simulink subsystem "pd_plus_controller_refsys"  (R2022b)
settings: Solver=VariableStepAuto  StartTime=0.0  StopTime=10.0  RelTol=1e-3
settings Model: Creator=emu  LastModifiedBy=emu

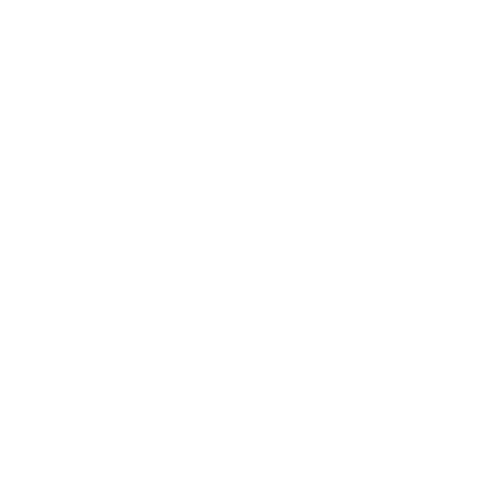
[thumbnail: Simulink's stored preview of the top-level diagram]
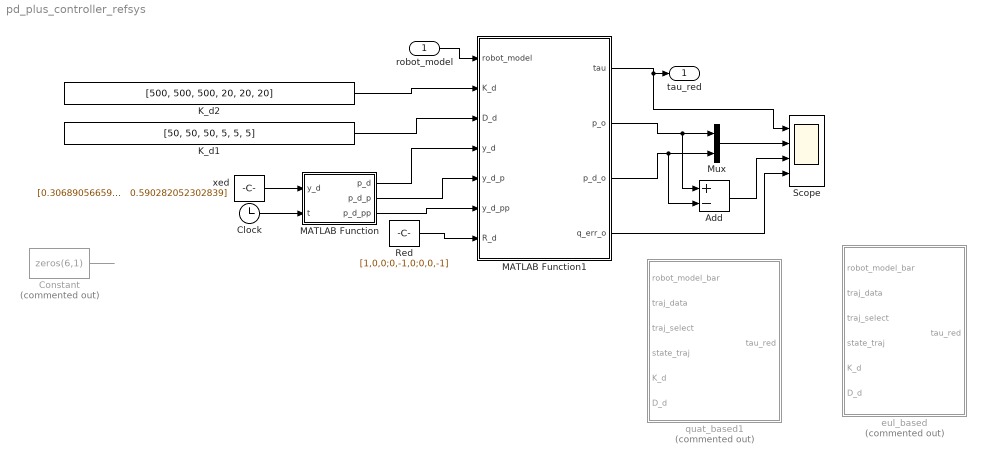
== system pd_plus_controller_refsys ==
  robot_model : Inport  OutDataTypeStr=Bus: robot_model_red
  Add : Sum  Inputs=+-
  Clock : Clock
  Constant : Constant  Commented=on  Value=zeros(6,1)
  K_d1 : Constant  Value=[50, 50, 50, 5, 5, 5]
  K_d2 : Constant  Value=[500, 500, 500, 20, 20, 20]
  MATLAB Function : MATLAB Function  TreatAsAtomicUnit=on
  MATLAB Function1 : MATLAB Function  TreatAsAtomicUnit=on
  Mux : Mux  Inputs=2
  Red : Constant  Value=[1,0,0;0,-1,0;0,0,-1]
  Scope : Scope  NumInputPorts=4
  eul_based : MATLAB Function  Commented=on  TreatAsAtomicUnit=on
  quat_based1 : MATLAB Function  Commented=on  TreatAsAtomicUnit=on
  xed : Constant  Value="[0.306890566592941  -0.000000000000000   0.590282052302839]"
  tau_red : Outport
  wires:
  robot_model/1 -> MATLAB Function1/1(robot_model)
  MATLAB Function1/1(tau) -> tau_red/1, Scope/1
  K_d2/1 -> MATLAB Function1/2(K_d)
  K_d1/1 -> MATLAB Function1/3(D_d)
  MATLAB Function/1(p_d) -> MATLAB Function1/4(y_d)
  Constant/1 -> ?
  MATLAB Function1/4(q_err_o) -> Scope/4
  Mux/1 -> Scope/2
  MATLAB Function1/2(p_o) -> Mux/1, Add/1
  MATLAB Function1/3(p_d_o) -> Mux/2, Add/2
  Clock/1 -> MATLAB Function/2(t)
  Red/1 -> MATLAB Function1/7(R_d)
  xed/1 -> MATLAB Function/1(y_d)
  MATLAB Function/2(p_d_p) -> MATLAB Function1/5(y_d_p)
  MATLAB Function/3(p_d_pp) -> MATLAB Function1/6(y_d_pp)
  Add/1 -> Scope/3

== matlab function pd_plus_controller_refsys/MATLAB Function ==
  data: y_d input; p_d output; t input; p_d_p output; p_d_pp output
function [p_d, p_d_p, p_d_pp] = fcn(y_d, t)

omega=0.1;
f = cos(omega*t);
df = -omega*sin(omega*t);
ddf = -omega^2 * cos(omega*t);

a=0.2;
p_d = [y_d(1); -0.2+y_d(2)+a*f; y_d(3)];
p_d_p = [0; a*df; 0];
p_d_pp = [0; a*ddf; 0];

== matlab function pd_plus_controller_refsys/MATLAB Function1 ==
  data: robot_model input Bus: robot_model_red; tau output; K_d input; D_d input; y_d input; y_d_p input; y_d_pp input; p_o output; p_d_o output; q_err_o output; R_d input
function [tau, p_o, p_d_o, q_err_o] = fcn(robot_model, K_d, D_d, y_d, y_d_p, y_d_pp, R_d)

M = robot_model.M;
C_rnea = robot_model.C_rnea;
J = robot_model.J;
J_p = robot_model.J_p;
H = robot_model.H;

q = robot_model.q;
q_p = robot_model.q_p;

% Desired Trajectory
p_d    = y_d;
p_d_p  = y_d_p;
p_d_pp = y_d_pp;

omega_d = zeros(3,1);
omega_d_p = zeros(3,1);

% Actual Sizes
x_p = J * q_p;
R = H(1:3,1:3);

p = H(1:3,4);
p_p = x_p(1:3);

omega = x_p(4:6); % Drehwinkelgeschwindigkeit des Endeffektors

% Errors
RR = R_d'*R;
q_err_tmp   = rotm2quat_v4(RR);
epsilon = q_err_tmp(2:4);
eta = q_err_tmp(1);
q_err = 2 * R_d * (eta * eye(3) + skew(epsilon)) * (K_d(4:6) .* epsilon);

x_err   = [K_d(1:3) .* (p-p_d); q_err];   % Error as quaternion
x_err_p = [p_p-p_d_p;  omega-omega_d];
x_d_pp  = [p_d_pp;     omega_d_p];

J_sym = J * J' + 1e-6*eye(6);
J_sym2 = 1/2 * (J_sym + J_sym');
J_pinv = J'/J_sym2;

tau = C_rnea + M*J_pinv*(x_d_pp - J_p*q_p) - J' * (D_d .* x_err_p + x_err);

p_o = p;
p_d_o = p_d;
q_err_o = q_err;

== matlab function pd_plus_controller_refsys/quat_based1 ==
  data: robot_model_bar input; tau_red output; traj_data input Bus: traj_data_bus; traj_select input; state_traj input Bus: state_traj_bus; K_d input; D_d input; param_robot parameter
function tau_red = fcn(robot_model_bar, traj_data, traj_select, state_traj, K_d, D_d, param_robot)

persistent cnt;
persistent run_flag;

if(isempty(cnt))
    cnt = 1;
    run_flag = 0;
end

%cnt = 1; % ignore cnt;

n_red = param_robot.n_red;
n_indices = param_robot.n_indices;

q_bar = robot_model_bar.q;
q_p_bar = robot_model_bar.q_p;

M_bar = robot_model_bar.M;
C_bar = robot_model_bar.C;
J_bar = robot_model_bar.J;
J_p_bar = robot_model_bar.J_p;
H_bar = robot_model_bar.H;

M_red = M_bar(n_indices, n_indices);
C_red = C_bar(n_indices, n_indices);
J_red = J_bar(:, n_indices);
J_p_red = J_p_bar(:, n_indices);

q_red = q_bar(n_indices);
q_p_red = q_p_bar(n_indices);

% Desired Trajectory
p_d    = traj_data.p_d(:, cnt, traj_select);
p_d_p  = traj_data.p_d_p(:, cnt, traj_select);
p_d_pp = traj_data.p_d_pp(:, cnt, traj_select);

R_d = traj_data.R_d(:, :, cnt, traj_select);
omega_d = traj_data.omega_d(:, cnt, traj_select);
omega_d_p = traj_data.omega_d_p(:, cnt, traj_select);

quat_d = traj_data.q_d(:, cnt, traj_select);
quat_d_p = traj_data.q_d_p(:, cnt, traj_select);
quat_d_pp = traj_data.q_d_pp(:, cnt, traj_select);

% Actual Sizes
x_p = J_red * q_p_red;
R = H_bar(1:3,1:3);

p = H_bar(1:3,4);
p_p = x_p(1:3);

omega = x_p(4:6); % Drehwinkelgeschwindigkeit des Endeffektors

Q = @(q) 0.5 * [ -q(2) -q(3) -q(4); ...
                  q(1)  q(4) -q(3); ...
                 -q(4)  q(1)  q(2); ...
                  q(3) -q(2)  q(1)];

quat = rotm2quat_v4(R);
quat = my_sign(quat(1))*quat;
quat_p = Q(quat)*omega;

J_omega = J_red(4:6,:);
J_omega_p = J_p_red(4:6,:);

J_quat = Q(quat)*J_omega;
J_quat_p = Q(quat_p)*J_omega + Q(quat)*J_omega_p;

J = [J_red(1:3,:);J_quat];
J_p = [J_p_red(1:3,:); J_quat_p];
%J_pinv = J\eye(7);

J_sym = J' * J + 1e-6*eye(6);
J_sym2 = 1/2 * (J_sym + J_sym');
J_pinv = J_sym2\J';

% Errors
RR = R_d'*R;
q_err_tmp   = rotm2quat_v4(RR);
epsilon = q_err_tmp(2:4);
eta = q_err_tmp(1);
q_err = 2 * R_d * (eta * eye(3) + skew(epsilon)) * (K_d(4:6) .* epsilon);

x_err   = [p-p_d;      quat - quat_d];   % Error as quaternion
x_err_p = [p_p-p_d_p;  quat_p-quat_d_p];
x_d_pp  = [p_d_pp;     quat_d_pp];

tau_red = C_red * q_p_red + M_red*J_pinv*(x_d_pp - J_p*q_p_red) - J' * (D_d .* x_err_p + K_d .* x_err);

[run_flag, cnt] = update_traj_cnt(state_traj, run_flag, cnt, traj_data.N);

end

function y = my_sign(x)
    y = (x >= 0)*2 - 1;
end

== matlab function pd_plus_controller_refsys/eul_based ==
  data: robot_model_bar input; tau_red output; traj_data input Bus: traj_data_bus; traj_select input; state_traj input Bus: state_traj_bus; K_d input; D_d input; param_robot parameter
function tau_red = fcn(robot_model_bar, traj_data, traj_select, state_traj, K_d, D_d, param_robot)

persistent cnt;
persistent run_flag;

if(isempty(cnt))
    cnt = 1;
    run_flag = 0;
end

%cnt = 1; % ignore cnt;

n_red = param_robot.n_red;
n_indices = param_robot.n_indices;

q_bar = robot_model_bar.q;
q_p_bar = robot_model_bar.q_p;

M_bar = robot_model_bar.M;
C_bar = robot_model_bar.C;
J_bar = robot_model_bar.J;
J_p_bar = robot_model_bar.J_p;
H_bar = robot_model_bar.H;

M_red = M_bar(n_indices, n_indices);
C_red = C_bar(n_indices, n_indices);
J_red = J_bar(:, n_indices);
J_p_red = J_p_bar(:, n_indices);

q_red = q_bar(n_indices);
q_p_red = q_p_bar(n_indices);

% Desired Trajectory
p_d    = traj_data.p_d(:, cnt, traj_select);
p_d_p  = traj_data.p_d_p(:, cnt, traj_select);
p_d_pp = traj_data.p_d_pp(:, cnt, traj_select);

phi_d = traj_data.Phi_d(:, cnt, traj_select);
phi_d_p = traj_data.Phi_d_p(:, cnt, traj_select);
phi_d_pp = traj_data.Phi_d_pp(:, cnt, traj_select);

R = H_bar(1:3,1:3);
phi = rotm2rpy(R);

T_mat = [eye(3), zeros(3); zeros(3), T_rpy(phi)];
J_a = T_mat\J_red;

x_p = J_a * q_p_red;
phi_p = x_p(4:6); % Drehwinkelgeschwindigkeit des Endeffektors

dT_mat = [zeros(3), zeros(3); zeros(3), T_rpy_p(phi, phi_p)];
J_a_p = T_mat\(J_p_red - dT_mat*J_a);

% Actual Sizes

p = H_bar(1:3,4);
p_p = x_p(1:3);

% Errors

x_err   = [p-p_d;      phi-phi_d];   % Error as quaternion
x_err_p = [p_p-p_d_p;  phi_p-phi_d_p];
x_d_pp  = [p_d_pp;     phi_d_pp];

J_pinv = J_a\eye(6);

tau_red = C_red * q_p_red + M_red*J_pinv*(x_d_pp - J_a_p*q_p_red) - J_a' * (D_d .* x_err_p + K_d .* x_err);

[run_flag, cnt] = update_traj_cnt(state_traj, run_flag, cnt, traj_data.N);
